simulink model "W3P3"  (R2020b)
settings: Solver=VariableStepAuto  StartTime=0.0  StopTime=10.0  RelTol=1e-3
values from neighbouring files (symbols this model uses):
  g = 9.81    [para.m]
  J = 0.01    [para.m]
  K = 1000    [para.m]
  m = 1200    [para.m]
  R = 0.28    [para.m]
  T = 0.01    [para.m]
  Tbmax = 2000    [para.m]
  V0 = 28    [para.m]
  Vmin = 1.4    [para.m]
settings Model: DataDictionary=week3prob3.sldd  Creator=HP  LastModifiedBy=HP

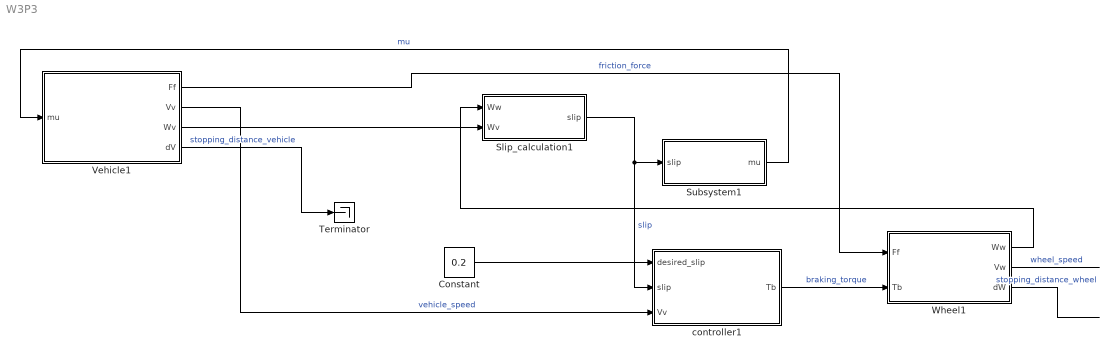
== system W3P3 ==
  Constant : Constant  Value=0.2
  Slip_calculation1 : Subsystem
  Subsystem1 : Subsystem
  Terminator : Terminator
  Vehicle1 : Subsystem
  Wheel1 : Subsystem
  controller1 : Subsystem
  wires:
  Wheel1/1(Ww) -> Slip_calculation1/1(Ww)
  Wheel1/3(dW) -> ?  "stopping_distance_wheel"
  Vehicle1/3(Wv) -> Slip_calculation1/2(Wv)
  controller1/1(Tb) -> Wheel1/2(Tb)  "braking_torque"
  Vehicle1/4(dV) -> Terminator/1  "stopping_distance_vehicle"
  Slip_calculation1/1(slip) -> controller1/2(slip), Subsystem1/1(slip)  "slip"
  Constant/1 -> controller1/1(desired_slip)
  Wheel1/2(Vw) -> ?  "wheel_speed"
  Vehicle1/2(Vv) -> controller1/3(Vv)  "vehicle_speed"
  Subsystem1/1(mu) -> Vehicle1/1(mu)  "mu"
  Vehicle1/1(Ff) -> Wheel1/1(Ff)  "friction_force"

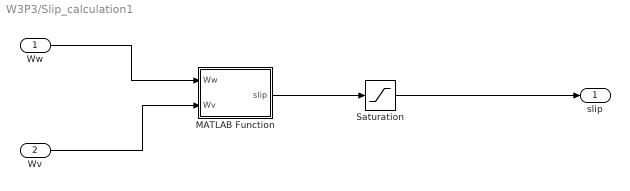
== system W3P3/Slip_calculation1 ==
  Ww : Inport
  Wv : Inport  Port=2
  MATLAB Function : MATLAB Function  TreatAsAtomicUnit=on
  Saturation : Saturate  UpperLimit=1  LowerLimit=0
  slip : Outport
  wires:
  Ww/1 -> MATLAB Function/1(Ww)
  Wv/1 -> MATLAB Function/2(Wv)
  MATLAB Function/1(slip) -> Saturation/1
  Saturation/1 -> slip/1

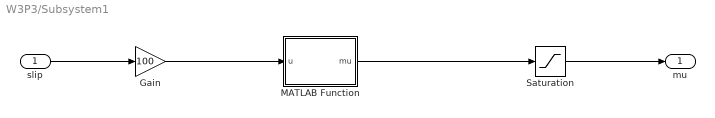
== system W3P3/Subsystem1 ==
  slip : Inport
  Gain : Gain  Gain=100
  MATLAB Function : MATLAB Function  TreatAsAtomicUnit=on
  Saturation : Saturate  UpperLimit=1  LowerLimit=0
  mu : Outport
  wires:
  Saturation/1 -> mu/1
  slip/1 -> Gain/1
  Gain/1 -> MATLAB Function/1(u)
  MATLAB Function/1(mu) -> Saturation/1

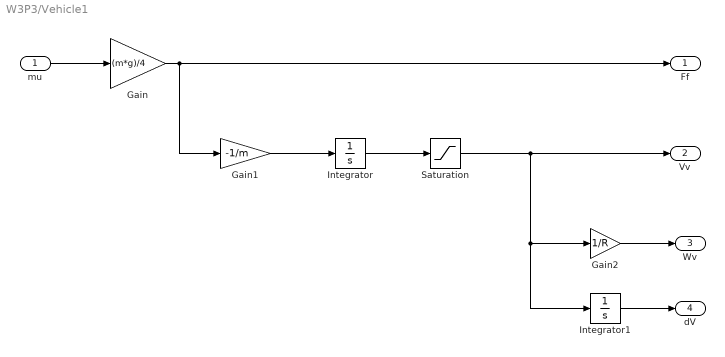
== system W3P3/Vehicle1 ==
  mu : Inport
  Gain : Gain  Gain=(m*g)/4
  Gain1 : Gain  Gain=-1/m
  Gain2 : Gain  Gain=1/R
  Integrator : Integrator  InitialCondition=V0
  Integrator1 : Integrator
  Saturation : Saturate  UpperLimit=1000  LowerLimit=0.001
  Ff : Outport
  Vv : Outport  Port=2
  Wv : Outport  Port=3
  dV : Outport  Port=4
  wires:
  mu/1 -> Gain/1
  Gain/1 -> Gain1/1, Ff/1
  Gain1/1 -> Integrator/1
  Integrator/1 -> Saturation/1
  Saturation/1 -> Integrator1/1, Gain2/1, Vv/1
  Gain2/1 -> Wv/1
  Integrator1/1 -> dV/1

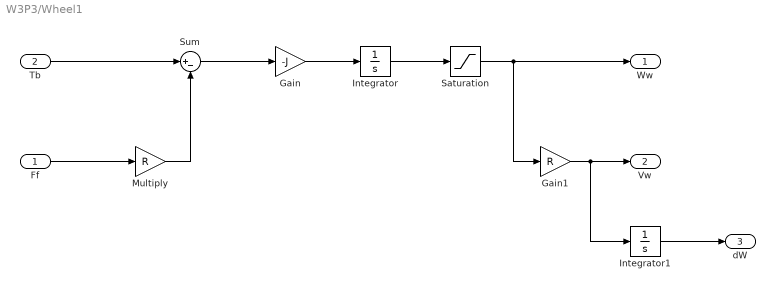
== system W3P3/Wheel1 ==
  Ff : Inport
  Tb : Inport  Port=2
  Gain : Gain  Gain=-J
  Gain1 : Gain  Gain=R
  Integrator : Integrator  InitialCondition=28/R
  Integrator1 : Integrator
  Multiply : Gain  Gain=R
  Saturation : Saturate  UpperLimit=1000  LowerLimit=0
  Sum : Sum  Inputs=|+-
  Ww : Outport
  Vw : Outport  Port=2
  dW : Outport  Port=3
  wires:
  Ff/1 -> Multiply/1
  Tb/1 -> Sum/1
  Multiply/1 -> Sum/2
  Sum/1 -> Gain/1
  Gain/1 -> Integrator/1
  Integrator/1 -> Saturation/1
  Saturation/1 -> Gain1/1, Ww/1
  Gain1/1 -> Integrator1/1, Vw/1
  Integrator1/1 -> dW/1

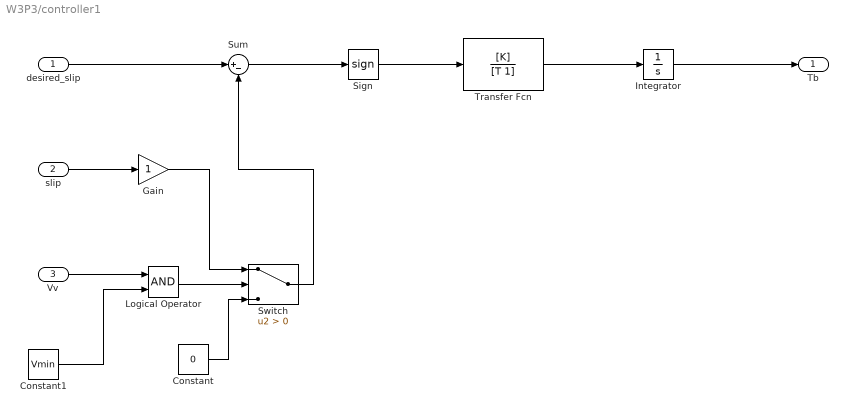
== system W3P3/controller1 ==
  desired_slip : Inport
  slip : Inport  Port=2
  Vv : Inport  Port=3
  Constant : Constant  Value=0
  Constant1 : Constant  Value=Vmin
  Gain : Gain
  Integrator : Integrator  LimitOutput=on  UpperSaturationLimit=Tbmax  LowerSaturationLimit=0
  Logical Operator : Logic  AllPortsSameDT=off  OutDataTypeStr=boolean
  Sign : Signum
  Sum : Sum  Inputs=|+-
  Switch : Switch  Criteria=u2 > Threshold
  Transfer Fcn : TransferFcn  Numerator=[K]  Denominator=[T 1]
  Tb : Outport
  wires:
  slip/1 -> Gain/1
  Vv/1 -> Logical Operator/1
  Logical Operator/1 -> Switch/2
  Integrator/1 -> Tb/1
  desired_slip/1 -> Sum/1
  Switch/1 -> Sum/2
  Constant/1 -> Switch/3
  Constant1/1 -> Logical Operator/2
  Gain/1 -> Switch/1
  Sum/1 -> Sign/1
  Sign/1 -> Transfer Fcn/1
  Transfer Fcn/1 -> Integrator/1

== matlab function W3P3/Subsystem1/MATLAB Function ==
  data: u input; mu output
function mu = fcn(u)

mu=0.7*(1.07*(1-exp(-0.5*u)-0.003*u));

== matlab function W3P3/Slip_calculation1/MATLAB Function ==
  data: Ww input; slip output; Wv input
function slip = fcn(Ww, Wv)

slip=1-(Ww/(Wv+(Wv==0)*eps));
